simulink model "DDADDT"  (R2024b)
settings: Solver=VariableStepAuto  StartTime=0.0  StopTime=10.0  RelTol=1e-3
libraries: simulink x1
settings Model: Creator=jaytinsley  LastModifiedBy=jaytinsley

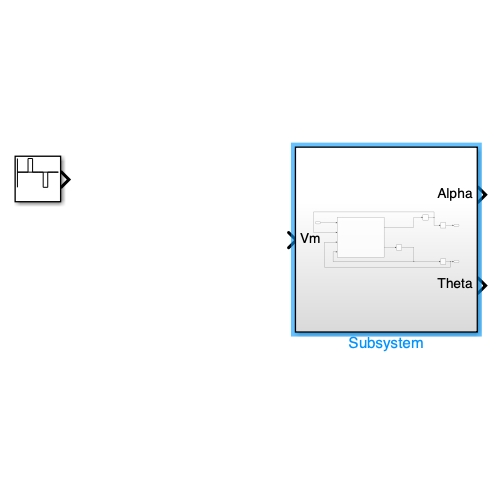
[thumbnail: Simulink's stored preview of the top-level diagram]
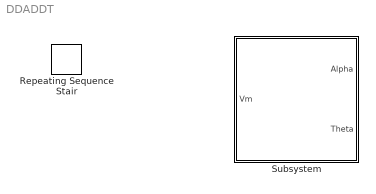
== system DDADDT ==
  Repeating Sequence Stair : simulink/Sources/Repeating Sequence Stair  OutValues=[0 0 1 0 0 -1 0 0]  tsamp=-1  OutMin=[]  OutMax=[]  OutDataTypeStr=double  OutputDataTypeScalingMode=double  OutDataType=fixdt(0,8)  ConRadixGroup=Best Precision: Vector-wise  OutScaling=2^-12
  Subsystem : Subsystem

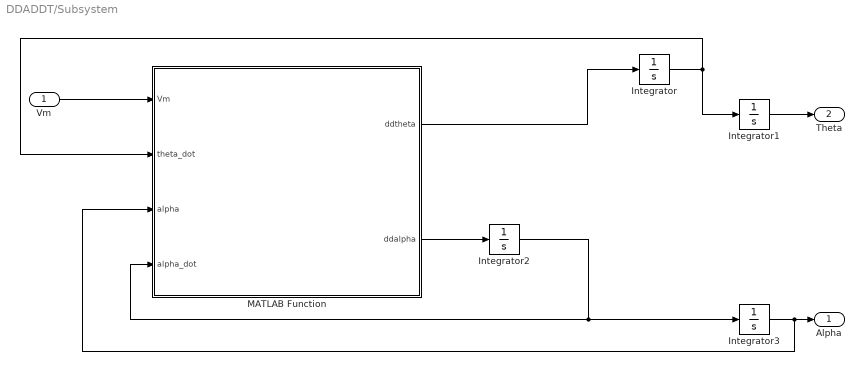
== system DDADDT/Subsystem ==
  Vm : Inport
  Integrator{,1..3} (4 alike) : Integrator
  MATLAB Function : MATLAB Function  TreatAsAtomicUnit=on
  Alpha : Outport
  Theta : Outport  Port=2
  wires:
  Vm/1 -> MATLAB Function/1(Vm)
  MATLAB Function/1(ddtheta) -> Integrator/1
  Integrator/1 -> Integrator1/1, MATLAB Function/2(theta_dot)
  Integrator1/1 -> Theta/1
  Integrator2/1 -> MATLAB Function/4(alpha_dot), Integrator3/1
  MATLAB Function/2(ddalpha) -> Integrator2/1
  Integrator3/1 -> MATLAB Function/3(alpha), Alpha/1

== matlab function DDADDT/Subsystem/MATLAB Function ==
  data: Vm input; theta_dot input; ddtheta output; alpha input; alpha_dot input; ddalpha output
function [ddtheta, ddalpha] = rp_dynamics_from_voltage(Vm, theta_dot, alpha, alpha_dot)
% Rotary pendulum dynamics solved concurrently using your given parameters.
% Inputs:
%   Vm         : motor voltage (V)
%   theta_dot  : rotary arm angular rate (rad/s)
%   alpha      : pendulum angle (rad)
%   alpha_dot  : pendulum angular rate (rad/s)
%   Dr, Dp     : viscous damping (N·m·s/rad) about rotary joint and pendulum joint
% Outputs:
%   ddtheta, ddalpha : angular accelerations (rad/s^2)

% ====== CONSTANTS (from your message) ======
V_nom = 18;
T_nom = 22.0*10^-3; %#ok<NASGU>
w_nom = 3050;      %#ok<NASGU> % (rpm?) not used here
I_nom = 0.540;     %#ok<NASGU>

R_m = 8.4;
k_t = 0.042;   % torque constant (N·m/A)
k_m = 0.042;   % back-EMF constant (V·s/rad)
J_m = 4.0e-6;  % motor rotor inertia (kg·m^2)
L_m = 1.16e-3; %#ok<NASGU> % armature inductance (not used in quasi-static tau)

m_h = 0.0106;
r_h = 0.0111;
J_h = 0.6e-6;

m_d = 0.053;
r_d = 0.0248;

% Rotary arm
m_r = 0.095;
L_r = 0.085;

% Pendulum link
m_p = 0.024;
L_p = 0.129;

g = 9.81;

Dr = 0.0015;

Dp = 0.0005;

% ====== INERTIAS (reasonable rigid-body approximations) ======
% Rotary side equivalent inertia about the pivot:
%  - motor rotor J_m
%  - hub disk J_h plus parallel-axis from hub mass m_h at radius r_h
%  - extra disk mass m_d at radius r_d
%  - slender arm of length L_r about one end: (1/3)*m_r*L_r^2
Jr = J_m + J_h + m_h*r_h^2 + m_d*r_d^2 + (1/3)*m_r*L_r^2;

% Pendulum slender rod about the joint:
Jp = (1/3)*m_p*L_p^2;

% ====== Motor torque (quasi-static electrical model) ======
% tau = k_t (V - k_m*theta_dot)/R_m
tau = k_t * (Vm - k_m*theta_dot) / R_m;

% ====== Dynamics (mass matrix and RHS) ======
A11 = m_p*L_r^2 + Jr;
A12 = -0.5*m_p*L_p*L_r;
A21 =  0.5*m_p*L_p*L_r;
A22 =  Jp + 0.25*m_p*L_p^2;

b1 =  tau - Dr*theta_dot;
b2 = -0.5*m_p*L_p*g*alpha - Dp*alpha_dot;

% Solve A * [ddtheta; ddalpha] = b
x = [A11, A12; A21, A22] \ [b1; b2];

ddtheta = x(1);
ddalpha = x(2);
end
